simulink model "AdaptiveandRRTxBackstepping21a"  (R2022a)
settings: Solver=ode1  StartTime=0.0  StopTime=30  FixedStep=0.01  RelTol=1e-3  EnableMultiTasking=on
undefined symbols (not defined in the file): ux, uy
libraries: arduinolib x5, arduinosensorlib x1, mobileRoboticsLib x1
(part 1 of 2)
settings Model: NumberOfSteps=10  ExtModeTrigDuration=2  Creator=TR  LastModifiedBy=LabPC
settings DataIOCC: ReturnWorkspaceOutputs=off
settings OptimizationCC: EnhancedBackFolding=on  PassReuseOutputArgsAs=Individual arguments  ZeroExternalMemoryAtStartup=off  ZeroInternalMemoryAtStartup=off  MaxStackSize=64  OptimizeBlockOrder=speed  DifferentSizesBufferReuse=on  OptimizationCustomize=off  EfficientTunableParamExpr=on
settings DebuggingCC: ParameterTunabilityLossMsg=error  UnconnectedInputMsg=warning  UnconnectedOutputMsg=warning  UnconnectedLineMsg=warning
settings HardwareCC: ProdBitPerPointer=32  ProdBitPerSizeT=32  ProdBitPerPtrDiffT=32  ProdLargestAtomicInteger=Long  ProdLargestAtomicFloat=Double  ProdWordSize=32  ProdHWDeviceType=ARM Compatible->ARM Cortex
settings SFSimCC: MATLABDynamicMemAlloc=off
settings RTWCC: SystemTargetFile=ert.tlc  HardwareBoard=Arduino Due  TemplateMakefile=ert_default_tmf  Toolchain=Arduino ARM  BuildConfiguration=Faster Runs  DLArmComputeVersion=19.05
settings CodeAppCC: ForceParamTrailComments=on  IgnoreCustomStorageClasses=off  OperatorAnnotations=on  SimulinkDataObjDesc=on  SFDataObjDesc=on  InsertBlockDesc=on
settings ERTTargetCC: SupportContinuousTime=on  SupportVariableSizeSignals=on  ExtMode=on  ExtModeTransport=3  ExtModeStaticAlloc=on  ExtModeStaticAllocSize=24576  ExtModeMexFile=ext_xcp  ExtModeMexArgs=0 3 115200  ExtModeIntrfLevel=Level2 - Open

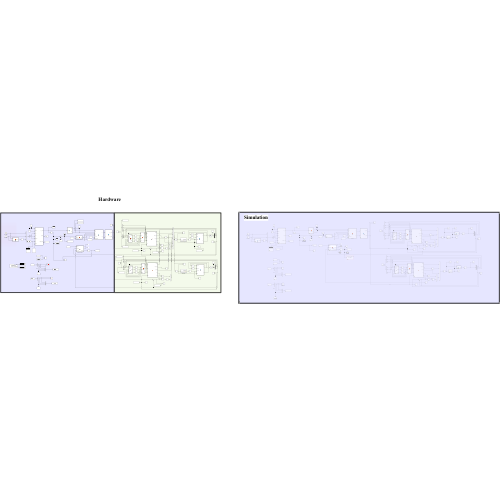
[thumbnail: Simulink's stored preview of the top-level diagram]
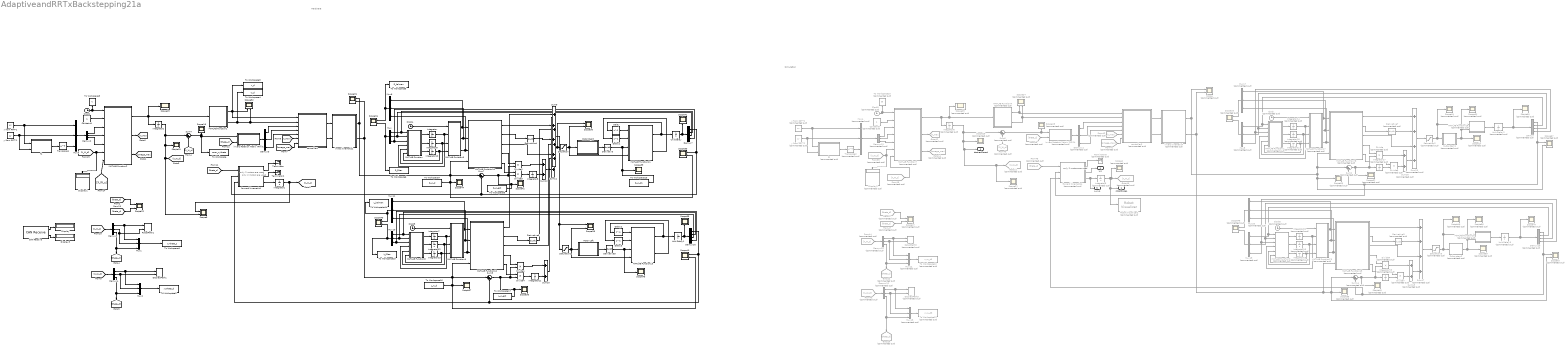
== system AdaptiveandRRTxBackstepping21a ==
  note: Hardware
  note: Simulation
  note: only 2 motors are used
  note: only 2 motors are used
  note: only 2 motors are used
  CAN Receive : arduinolib/CAN Receive  outputDataType=Raw data  identifierType=Standard (11-bit identifier)  messageId=100  msgLength=8  SampleTime=0.01  outputError=off  outputRemote=off
      settings: SourceProductBaseCode=ARDUINO
  Clock : Clock  Commented=on
  Clock1 : Clock
  Clock3 : Clock  Commented=on
  Clock4 : Clock
  Clock5 : Clock
  Clock6 : Clock  Commented=on
  Constant1 : Constant
  Constant2 : Constant  Commented=on
  Delay : Delay  DelayLength=1  InitialCondition=[0;0;0;0]
  Delay1 : Delay  DelayLength=1  InitialCondition=1e0*diag([10,1,30,10])
  Delay2 : Delay  DelayLength=1  InitialCondition=[0;0;0;0]
  Delay3 : Delay  DelayLength=1  InitialCondition=1e0*diag([10,1,30,10])
  Demux : Demux  Commented=on
  Demux{10..13} (4 alike) : Demux  Commented=on  Outputs=3
  Demux16 : Demux
  Demux{2..5} (4 alike) : Demux  Outputs=3
  Demux20 : Demux  Commented=on
  Demux7 : Demux
  Derivative{,4..6} (4 alike) : Derivative
  Derivative3 : Derivative  Commented=on
  Derivative7 : Derivative  Commented=on
  DesiredPath1 : Record  FileSettingsInternal="{\"entries\":[{\"content\":{\"excelSettings\":{\"content\":{},\"type\":\"Streamout.ExcelSettings\"}},\"type\":\"Streamout.FileSettingStorage\",\"uuid\":\"4478c04d-78d5-4c1c-a069-eeebce6a06e9\"}],\"packageUris\":[\"http://schema.mathworks.com/mf0/streamout_blocks/R2020a\"],\"version\":\"1.0\"}"  Layout=[1 1]  SignalsInternal="{\"entries\":[{\"content\":{\"signals\":[{\"content\":{\"blockPath\":[\"AdaptiveandRRTxBackstepping21a/DesiredPath1\"],\"channel\":[],\"dimensions\":[1],\"domain\":\"AdaptiveandRRTxBackstepping21a/DesiredPath1\",\"lineColor\":\"#a2142f\",\"plots\":[1],\"port\":1,\"sid\":[],\"signalID\":57046,\"signalName\":\"Demux4:1\"},\"type\":\"RecordBlkView.Signal\",\"uuid\":\"8b54ff27-c98d-4d9d-9907-af57662ca3f3\"},{\"content\":{\"blockPath\":[\"AdaptiveandRRTxBackstepping21a/DesiredPath1\"],\"channel\":[],\"dimensions\":[1],\"domain\":\"AdaptiveandRRTxBackstepping21a/DesiredPath1\",\"lineColor\":\"#139fff\",\"plots\":[1],\"port\":2,\"sid\":[],\"signalID\":57049,\"signalName\":\"Demux4:2\"},\"type\":\"RecordBlkView.Signal\",\"uuid\":\"d182928c-e909-4326-8931-a59e582ad6a8\"}]},\"type\":\"RecordBlkView.InputSignals\",\"uuid\":\"9f6ffbd3-a541-4e0a-a157-84b9438781ea\"}],\"packageUris\":[\"http://schema.mathworks.com/mf0/streamout_blocks/R2020a\"],\"version\":\"1.0\"}"  VisualizationBindings="{\"xyplotplugin\":{\"info\":[{\"series\":[{\"bindingParametersList\":[{\"parameter\":\"X-Axis\",\"signalID\":57046,\"signalName\":\"Demux4:1\"},{\"parameter\":\"Y-Axis\",\"signalID\":57049,\"signalName\":\"Demux4:2\"}],\"seriesID\":54754}],\"subplotID\":1}]}}"  CompatibilityTag=XY  st=-1
  DesiredPath3 : Record  Commented=on  FileSettingsInternal="{\"entries\":[{\"content\":{\"excelSettings\":{\"content\":{},\"type\":\"Streamout.ExcelSettings\"}},\"type\":\"Streamout.FileSettingStorage\",\"uuid\":\"5e9f582f-be01-4ee5-aef2-fee70209bf0f\"}],\"packageUris\":[\"http://schema.mathworks.com/mf0/streamout_blocks/R2020a\"],\"version\":\"1.0\"}"  Layout=[1 1]  SignalsInternal="{\"entries\":[{\"content\":{\"signals\":[{\"content\":{\"blockPath\":[\"AdaptiveandRRTxBackstepping21a/DesiredPath3\"],\"channel\":[],\"dimensions\":[1],\"domain\":\"AdaptiveandRRTxBackstepping21a/DesiredPath3\",\"lineColor\":\"#a2142f\",\"plots\":[1],\"port\":1,\"sid\":[],\"signalID\":57038,\"signalName\":\"XY Graph:1\"},\"type\":\"RecordBlkView.Signal\",\"uuid\":\"5ec44264-e469-460e-9c8e-a5441ec41171\"},{\"content\":{\"blockPath\":[\"AdaptiveandRRTxBackstepping21a/DesiredPath3\"],\"channel\":[],\"dimensions\":[1],\"domain\":\"AdaptiveandRRTxBackstepping21a/DesiredPath3\",\"lineColor\":\"#139fff\",\"plots\":[1],\"port\":2,\"sid\":[],\"signalID\":57041,\"signalName\":\"XY Graph:2\"},\"type\":\"RecordBlkView.Signal\",\"uuid\":\"ca682f9e-4f20-4675-ba71-c6bfc3bf3438\"}]},\"type\":\"RecordBlkView.InputSignals\",\"uuid\":\"5794ffc7-f7ba-41dc-b1e7-413d37048635\"}],\"packageUris\":[\"http://schema.mathworks.com/mf0/streamout_blocks/R2020a\"],\"version\":\"1.0\"}"  VisualizationBindings="{\"xyplotplugin\":{\"info\":[{\"series\":[{\"bindingParametersList\":[{\"parameter\":\"X-Axis\",\"signalID\":57038,\"signalName\":\"XY Graph:1\"},{\"parameter\":\"Y-Axis\",\"signalID\":57041,\"signalName\":\"XY Graph:2\"}],\"seriesID\":2614}],\"subplotID\":1}]}}"  CompatibilityTag=XY  st=-1
  Display : Display
  Display1 : Display
  Display2 : Display  Commented=on
  Display3 : Display
  Divide{,5..7} (4 alike) : Product  Commented=on  Inputs=**
  Divide{1..4} (4 alike) : Product  Inputs=**
  From15 : From  Commented=on  GotoTag=X_W_c
  From35 : From  Commented=on  GotoTag=X_W_d
  From37 : From  Commented=on  GotoTag=theta_d
  From40 : From  Commented=on  GotoTag=X_W_c
  From41 : From  Commented=on  GotoTag=omega_max
  From42 : From  Commented=on  GotoTag=V_max
  From43 : From  Commented=on  GotoTag=X_W_d
  From44 : From  Commented=on  GotoTag=X_W_c
  From45 : From  Commented=on  GotoTag=theta_c
  From46 : From  Commented=on  GotoTag=theta_c
  From47 : From  Commented=on  GotoTag=theta_c
  Goto12 : Goto  Commented=on  GotoTag=V_max
  Goto14 : Goto  Commented=on  GotoTag=omega_max
  Goto16 : Goto  Commented=on  GotoTag=X_W_c
  Goto21 : Goto  Commented=on  GotoTag=X_W_d
  Goto22 : Goto  Commented=on  GotoTag=theta_c
  Goto23 : Goto  Commented=on  GotoTag=theta_d
  Integrator : Integrator  InitialCondition=28.37
  Integrator1 : Integrator  InitialCondition=[0;0;0]
  Integrator10 : Integrator  InitialCondition=5.750
  Integrator11 : Integrator
  Integrator12 : Integrator  InitialCondition=17.26
  Integrator13 : Integrator  InitialCondition=6.776
  Integrator14 : Integrator  Commented=on  InitialCondition=28.37
  Integrator15 : Integrator  Commented=on  InitialCondition=17.26
  Integrator16 : Integrator  Commented=on  InitialCondition=6.776
  Integrator17 : Integrator  Commented=on
  Integrator18 : Integrator  Commented=on  InitialCondition=19.15
  Integrator2 : Integrator
  Integrator21 : Integrator  Commented=on  InitialCondition=5.75
  Integrator22 : Integrator  Commented=on  InitialCondition=26.63
  Integrator23 : Integrator  Commented=on
  Integrator5 : Integrator  Commented=on  InitialCondition=[0;0;0]
  Integrator6 : Integrator  Commented=on
  Integrator7 : Integrator  InitialCondition=26.63
  Integrator8 : Integrator
  Integrator9 : Integrator  InitialCondition=19.15
  MATLAB Function : MATLAB Function  TreatAsAtomicUnit=on
  MATLAB Function1 : MATLAB Function  TreatAsAtomicUnit=on
  MATLAB Function10 : MATLAB Function  TreatAsAtomicUnit=on
  MATLAB Function11 : MATLAB Function  TreatAsAtomicUnit=on
  MATLAB Function12 : MATLAB Function  TreatAsAtomicUnit=on
  MATLAB Function13 : MATLAB Function  TreatAsAtomicUnit=on
  MATLAB Function14 : MATLAB Function  Commented=on  TreatAsAtomicUnit=on
  MATLAB Function15 : MATLAB Function  Commented=on  TreatAsAtomicUnit=on
  MATLAB Function16 : MATLAB Function  Commented=on  TreatAsAtomicUnit=on
  MATLAB Function17 : MATLAB Function  Commented=on  TreatAsAtomicUnit=on
  MATLAB Function18 : MATLAB Function  Commented=on  TreatAsAtomicUnit=on
  MATLAB Function19 : MATLAB Function  Commented=on  TreatAsAtomicUnit=on
  MATLAB Function2 : MATLAB Function  TreatAsAtomicUnit=on
  MATLAB Function22 : MATLAB Function  Commented=on  TreatAsAtomicUnit=on
  MATLAB Function23 : MATLAB Function  Commented=on  TreatAsAtomicUnit=on
  MATLAB Function5 : MATLAB Function  TreatAsAtomicUnit=on
  MATLAB Function6 : MATLAB Function  Commented=on  TreatAsAtomicUnit=on
  MATLAB Function7 : MATLAB Function  Commented=on  TreatAsAtomicUnit=on
  MATLAB Function8 : MATLAB Function  TreatAsAtomicUnit=on
  MATLAB Function9 : MATLAB Function  TreatAsAtomicUnit=on
  Motor Left : Subsystem
  Motor Right : Subsystem
  Mux{,1..2,8..11} (7 alike) : Mux  Inputs=3
  Mux{4..5,12..13,17,19..20} (7 alike) : Mux  Commented=on  Inputs=3
  Robot Visualizer1 : mobileRoboticsLib/Environments/Robot Visualizer  Priority=99  Commented=on  robotRadius=0.22  showTrajectory=on  hasWaypoints=off  hasLidar=off  sensorOffset=scanSensorOffset  scanAngles=scanAngles  hasObjDetector=off  objDetectorOffset=[ 0, 0 ]  objDetectorAngle=0  objDetectorFOV=0  objDetectorMaxRange=0  objectColors=0  objectMarkers='s'
  RobotPath1 : Record  FileSettingsInternal="{\"entries\":[{\"content\":{\"excelSettings\":{\"content\":{},\"type\":\"Streamout.ExcelSettings\"}},\"type\":\"Streamout.FileSettingStorage\",\"uuid\":\"0ff43101-e007-4439-8427-ec14aa2ad80f\"}],\"packageUris\":[\"http://schema.mathworks.com/mf0/streamout_blocks/R2020a\"],\"version\":\"1.0\"}"  Layout=[1 1]  SignalsInternal="{\"entries\":[{\"content\":{\"signals\":[{\"content\":{\"blockPath\":[\"AdaptiveandRRTxBackstepping21a/RobotPath1\"],\"channel\":[],\"dimensions\":[1],\"domain\":\"AdaptiveandRRTxBackstepping21a/RobotPath1\",\"lineColor\":\"#a2142f\",\"plots\":[1],\"port\":1,\"sid\":[],\"signalID\":57030,\"signalName\":\"x_c\"},\"type\":\"RecordBlkView.Signal\",\"uuid\":\"07d52e62-8ab4-4c53-9fa3-f17bd603cef6\"},{\"content\":{\"blockPath\":[\"AdaptiveandRRTxBackstepping21a/RobotPath1\"],\"channel\":[],\"dimensions\":[1],\"domain\":\"AdaptiveandRRTxBackstepping21a/RobotPath1\",\"lineColor\":\"#139fff\",\"plots\":[1],\"port\":2,\"sid\":[],\"signalID\":57033,\"signalName\":\"y_c\"},\"type\":\"RecordBlkView.Signal\",\"uuid\":\"97726e5f-6405-4899-84cb-06a72cfc2d61\"}]},\"type\":\"RecordBlkView.InputSignals\",\"uuid\":\"38ea1586-2402-407b-8988-e549c318f5ad\"}],\"packageUris\":[\"http://schema.mathworks.com/mf0/streamout_blocks/R2020a\"],\"version\":\"1.0\"}"  VisualizationBindings="{\"xyplotplugin\":{\"info\":[{\"series\":[{\"bindingParametersList\":[{\"parameter\":\"X-Axis\",\"signalID\":57030,\"signalName\":\"x_c\"},{\"parameter\":\"Y-Axis\",\"signalID\":57033,\"signalName\":\"y_c\"}],\"seriesID\":57420}],\"subplotID\":1}]}}"  CompatibilityTag=XY  st=-1
  RobotPath3 : Record  Commented=on  FileSettingsInternal="{\"entries\":[{\"content\":{\"excelSettings\":{\"content\":{},\"type\":\"Streamout.ExcelSettings\"}},\"type\":\"Streamout.FileSettingStorage\",\"uuid\":\"6211d518-7cd9-4385-8e1e-1901f1a620c4\"}],\"packageUris\":[\"http://schema.mathworks.com/mf0/streamout_blocks/R2020a\"],\"version\":\"1.0\"}"  Layout=[1 1]  SignalsInternal="{\"entries\":[{\"content\":{\"signals\":[{\"content\":{\"blockPath\":[\"AdaptiveandRRTxBackstepping21a/RobotPath3\"],\"channel\":[],\"dimensions\":[1],\"domain\":\"AdaptiveandRRTxBackstepping21a/RobotPath3\",\"lineColor\":\"#a2142f\",\"plots\":[1],\"port\":1,\"sid\":[],\"signalID\":57022,\"signalName\":\"XY Graph:1\"},\"type\":\"RecordBlkView.Signal\",\"uuid\":\"6d308a3b-99d3-4536-8b9f-580f0f8d7449\"},{\"content\":{\"blockPath\":[\"AdaptiveandRRTxBackstepping21a/RobotPath3\"],\"channel\":[],\"dimensions\":[1],\"domain\":\"AdaptiveandRRTxBackstepping21a/RobotPath3\",\"lineColor\":\"#139fff\",\"plots\":[1],\"port\":2,\"sid\":[],\"signalID\":57025,\"signalName\":\"XY Graph:2\"},\"type\":\"RecordBlkView.Signal\",\"uuid\":\"215d46f4-e3f5-46fc-8db7-d861b213b18e\"}]},\"type\":\"RecordBlkView.InputSignals\",\"uuid\":\"501962c1-ec9d-432a-b496-bf00d34232ec\"}],\"packageUris\":[\"http://schema.mathworks.com/mf0/streamout_blocks/R2020a\"],\"version\":\"1.0\"}"  VisualizationBindings="{\"xyplotplugin\":{\"info\":[{\"series\":[{\"bindingParametersList\":[{\"parameter\":\"X-Axis\",\"signalID\":57022,\"signalName\":\"XY Graph:1\"},{\"parameter\":\"Y-Axis\",\"signalID\":57025,\"signalName\":\"XY Graph:2\"}],\"seriesID\":23653}],\"subplotID\":1}]}}"  CompatibilityTag=XY  st=-1
  Saturation : Saturate  UpperLimit=23  LowerLimit=-23
  Saturation1 : Saturate  UpperLimit=23  LowerLimit=-23
  Saturation2 : Saturate  Commented=on  UpperLimit=23  LowerLimit=-23
  Saturation3 : Saturate  Commented=on  UpperLimit=23  LowerLimit=-23
  Scope{,20..21,24,46,61..62} (7 alike) : Scope  Commented=on  NumInputPorts=2
  Scope{15,18..19,35..37,39,41..42,44..45} (11 alike) : Scope
  Scope{2,17,23,25,28..29,47..49,55..56,59..60,63..66} (17 alike) : Scope  Commented=on
  Scope{8,22,30..34,38,40,43} (10 alike) : Scope  NumInputPorts=2
  Subsystem1 : Subsystem  Commented=on
  Subsystem2 : Subsystem  Commented=on
  Sum10 : Sum
  Sum11 : Sum  Inputs=++++
  Sum12 : Sum
  Sum13 : Sum  Commented=on  Inputs=++++
  Sum14 : Sum  Commented=on  Inputs=|+-
  Sum16 : Sum  Commented=on
  Sum17 : Sum  Commented=on  Inputs=++++
  Sum18 : Sum  Commented=on
  Sum2 : Sum  Commented=on  Inputs=|+-
  Sum4 : Sum  Inputs=|+-
  Sum6 : Sum  Commented=on  Inputs=|+-
  Sum7 : Sum  Inputs=|+-
  Sum8 : Sum  Inputs=|+-
  Sum9 : Sum  Inputs=++++
  Terminator : Terminator
  Terminator1 : Terminator
  Terminator3 : Terminator  Commented=on
  To Workspace : ToWorkspace  VariableName=error_xytheta  SaveFormat=Structure With Time  SampleTime=-1
  To Workspace1 : ToWorkspace  VariableName=xytheta_c  SaveFormat=Structure With Time  SampleTime=-1
  To Workspace10 : ToWorkspace  Commented=on  VariableName=t3  SampleTime=-1
  To Workspace11 : ToWorkspace  Commented=on  VariableName=xyw_d3  SaveFormat=Timeseries  SampleTime=-1
  To Workspace12 : ToWorkspace  Commented=on  VariableName=xyw_c3  SaveFormat=Timeseries  SampleTime=-1
  To Workspace13 : ToWorkspace  VariableName=R_w_d1  SaveFormat=Structure With Time  SampleTime=-1
  To Workspace14 : ToWorkspace  VariableName=L_kalman  SaveFormat=Structure With Time  SampleTime=-1
  To Workspace15 : ToWorkspace  VariableName=L_filter  SaveFormat=Structure With Time  SampleTime=-1
  To Workspace16 : ToWorkspace  VariableName=L_w_d  SaveFormat=Structure With Time  SampleTime=-1
  To Workspace17 : ToWorkspace  VariableName=L_w_est  SaveFormat=Structure With Time  SampleTime=-1
  To Workspace2 : ToWorkspace  VariableName=xytheta_d  SaveFormat=Structure With Time  SampleTime=-1
  To Workspace3 : ToWorkspace  VariableName=v_d  SaveFormat=Structure With Time  SampleTime=-1
  To Workspace4 : ToWorkspace  VariableName=w_d  SaveFormat=Structure With Time  SampleTime=-1
  To Workspace5 : ToWorkspace  VariableName=R_kalman  SaveFormat=Structure With Time  SampleTime=-1
  To Workspace6 : ToWorkspace  VariableName=R_filter  SaveFormat=Structure With Time  SampleTime=-1
  To Workspace7 : ToWorkspace  VariableName=R_w_d  SaveFormat=Structure With Time  SampleTime=-1
  To Workspace8 : ToWorkspace  VariableName=R_w_est  SaveFormat=Structure With Time  SampleTime=-1
  To Workspace9 : ToWorkspace  VariableName=t  SampleTime=-1
  Transpose1 : Math  Operator=transpose
  Transpose2 : Math  Commented=on  Operator=transpose
  Unit Delay : UnitDelay  SampleTime=-1  HasFrameUpgradeWarning=on
  Unit Delay1 : UnitDelay  SampleTime=-1  HasFrameUpgradeWarning=on
  Unit Delay2 : UnitDelay  Commented=on  SampleTime=-1  HasFrameUpgradeWarning=on
  Unit Delay3 : UnitDelay  Commented=on  SampleTime=-1  HasFrameUpgradeWarning=on
  controller1 : MATLAB Function  TreatAsAtomicUnit=on
  controller3 : MATLAB Function  Commented=on  TreatAsAtomicUnit=on
  f1 : MATLAB Function  TreatAsAtomicUnit=on
  f2 : MATLAB Function  Commented=on  TreatAsAtomicUnit=on
  forward kinematic1 : MATLAB Function  TreatAsAtomicUnit=on
  forward kinematic4 : MATLAB Function  Commented=on  TreatAsAtomicUnit=on
  invers Rotation Matrix (R(fi))1 : MATLAB Function  TreatAsAtomicUnit=on
  invers Rotation Matrix (R(fi))4 : MATLAB Function  Commented=on  TreatAsAtomicUnit=on
  invers kinematic1 : MATLAB Function  TreatAsAtomicUnit=on
  invers kinematic4 : MATLAB Function  Commented=on  TreatAsAtomicUnit=on
  x from RRT*1 : Constant  Value=ux
  x from RRT*2 : Constant  Commented=on  Value=ux
  y from RRT*1 : Constant  Value=uy
  y from RRT*2 : Constant  Commented=on  Value=uy
  robotPose4 : Outport
  desiredPose4 : Outport  Port=2
  v_xy4 : Outport  Port=3
  w4 : Outport  Port=4
  wires:
  Demux11/1 -> controller3/3(e1)
  invers Rotation Matrix (R(fi))4/1(e_R) -> Demux11/1
  From41/1 -> controller3/7(omega_max)
  Mux4/1 -> Demux10/1
  Demux10/1 -> MATLAB Function7/3(x_d)
  MATLAB Function7/3(omega_max) -> Goto14/1
  From42/1 -> controller3/6(V_max)
  Demux10/3 -> MATLAB Function7/5(theta_d)
  MATLAB Function7/2(V_max) -> Goto12/1
  From40/1 -> Sum6/2  "xyd_c"
  Demux13/3 -> Mux12/3, Goto22/1  "theta_c"
  From37/1 -> Scope21/1
  controller3/2(w_c) -> invers kinematic4/2(w)
  MATLAB Function6/1(v_d) -> Scope24/1, controller3/1(v_d)
  Demux12/2 -> Mux13/2, DesiredPath3/2
  Demux10/2 -> MATLAB Function7/4(y_d)
  Integrator5/1 -> Scope2/1, Goto16/1, Robot Visualizer1/1, robotPose4/1
  Sum6/1 -> invers Rotation Matrix (R(fi))4/1(e_w), Scope28/1
  Demux12/1 -> Mux13/1, DesiredPath3/1
  y from RRT*2/1 -> Mux4/2, f2/2(y_d)
  Transpose2/1 -> Mux4/3
  Demux11/3 -> controller3/5(e3)
  Clock3/1 -> MATLAB Function7/1(t), To Workspace10/1
  Demux11/2 -> controller3/4(e2)
  From44/1 -> Demux13/1
  Mux13/1 -> To Workspace11/1
  Integrator6/1 -> Goto21/1, Scope23/1, desiredPose4/1, Scope29/1, Sum6/1  "xyw_d"
  Constant2/1 -> MATLAB Function7/2(route)
  forward kinematic4/2(w) -> w4/1
  From45/1 -> forward kinematic4/1(theta_c)
  x from RRT*2/1 -> f2/1(x_d), Mux4/1
  MATLAB Function7/1(X_r_dot) -> Scope25/1, MATLAB Function6/1(Xd_dot), Integrator6/1
  From35/1 -> Display2/1, MATLAB Function7/6(X)
  forward kinematic4/3(X_W_dot) -> Integrator5/1, v_xy4/1
  forward kinematic4/1(v) -> Terminator3/1
  From47/1 -> Scope21/2
  Demux13/2 -> Mux12/2, RobotPath3/2  "y_c"
  Demux13/1 -> Mux12/1, RobotPath3/1  "x_c"
  From46/1 -> invers Rotation Matrix (R(fi))4/2(theta_c)
  From43/1 -> Demux12/1
  Demux12/3 -> Goto23/1, Mux13/3  "theta_d"
  controller3/1(v_c) -> invers kinematic4/1(v)
  MATLAB Function6/2(w_d) -> controller3/2(w_d), Scope24/2
  f2/1(theta_d) -> Transpose2/1
  Mux12/1 -> To Workspace12/1
  From15/1 -> MATLAB Function7/7(X_W_c)
  Sum4/1 -> To Workspace/1, invers Rotation Matrix (R(fi))1/1(e_w), Scope18/1
  Demux2/1 -> MATLAB Function2/3(x_d)
  invers Rotation Matrix (R(fi))1/1(e_R) -> Demux3/1
  Demux5/1 -> Mux1/1, RobotPath1/1  "x_c"
  Demux4/2 -> DesiredPath1/2, Mux2/2
  [omega_max] -> controller1/7(omega_max)
  MATLAB Function2/3(omega_max) -> [omega_max]
  [theta_c] -> forward kinematic1/1(theta_c)
  [theta_d] -> Scope22/1
  Demux5/3 -> [theta_c], Mux1/3  "theta_c"
  controller1/2(w_c) -> invers kinematic1/2(w)
  Demux7/1 -> Sum7/2, forward kinematic1/2(fi_R_dot), Scope33/1
  Demux2/3 -> MATLAB Function2/5(theta_d)
  Integrator1/1 -> Scope8/1, [X_W_c]
  Demux4/1 -> DesiredPath1/1, Mux2/1
  MATLAB Function2/2(V_max) -> [V_max]
  Demux3/3 -> controller1/5(e3)
  [X_W_c] -> Sum4/2  "xyd_c"
  Mux9/1 -> Demux2/1
  Demux3/1 -> controller1/3(e1)
  Constant1/1 -> MATLAB Function2/2(route)
  forward kinematic1/1(v) -> Terminator/1
  forward kinematic1/3(X_W_dot) -> Integrator1/1
  MATLAB Function1/2(w_d) -> controller1/2(w_d), Scope32/2, To Workspace4/1
  x from RRT*1/1 -> Mux9/1, f1/1(x_d)
  MATLAB Function1/1(v_d) -> Scope32/1, To Workspace3/1, controller1/1(v_d)
  f1/1(theta_d) -> Transpose1/1
  Mux2/1 -> To Workspace2/1
  MATLAB Function2/1(X_r_dot) -> Scope15/1, Integrator2/1, MATLAB Function1/1(Xd_dot)
  Clock1/1 -> To Workspace9/1, MATLAB Function2/1(t)
  Demux3/2 -> controller1/4(e2)
  [V_max] -> controller1/6(V_max)
  Demux2/2 -> MATLAB Function2/4(y_d)
  forward kinematic1/2(w) -> Terminator1/1
  Mux1/1 -> To Workspace1/1
  [theta_c] -> Scope22/2
  Integrator2/1 -> Scope8/2, [X_W_d], Scope19/1, Sum4/1  "xyw_d"
  [X_W_c] -> MATLAB Function2/7(X_W_c)
  [X_W_d] -> Display1/1, MATLAB Function2/6(X)
  [theta_c] -> invers Rotation Matrix (R(fi))1/2(theta_c)
  y from RRT*1/1 -> f1/2(y_d), Mux9/2
  Demux4/3 -> Mux2/3, [theta_d]  "theta_d"
  controller1/1(v_c) -> invers kinematic1/1(v)
  Demux5/2 -> RobotPath1/2, Mux1/2  "y_c"
  [X_W_d] -> Demux4/1
  Transpose1/1 -> Mux9/3
  [X_W_c] -> Demux5/1
  MATLAB Function10/3(a_on_b) -> Sum11/3
  Derivative5/1 -> Scope45/1, MATLAB Function13/3(y_true)
  MATLAB Function9/1(a) -> Mux11/1, MATLAB Function12/1(a)
  Integrator7/1 -> MATLAB Function9/2(a_nw), MATLAB Function8/4(a)
  Derivative/1 -> To Workspace13/1, Scope39/1, MATLAB Function11/3(y_true)
  MATLAB Function5/1(a) -> Mux8/1, MATLAB Function10/1(a)
  Clock5/1 -> MATLAB Function9/1(t)
  Integrator12/1 -> MATLAB Function8/5(b), MATLAB Function9/3(b_nw)
  Divide1/1 -> Sum10/1
  Sum10/1 -> Sum9/4
  MATLAB Function12/5(ki) -> Divide4/1
  Saturation/1 -> MATLAB Function11/4(uk), Motor Right/1(u), Scope30/2
  invers kinematic1/1(fi_R_dot) -> MATLAB Function10/4(w), Scope44/1, To Workspace7/1, Scope33/2, Sum7/1, Scope31/1
  Sum9/1 -> Saturation1/1, Scope38/1
  Unit Delay1/1 -> Demux16/1, Scope35/1
  Demux7/3 -> MATLAB Function/2(b_hat), Mux/2
  MATLAB Function12/1(comp) -> Sum9/1
  MATLAB Function13/1(x) -> Delay2/1, Unit Delay1/1
  Demux16/3 -> MATLAB Function8/2(b_hat), Mux10/2
  invers kinematic1/2(fi_L_dot) -> Scope31/2, Scope40/2, To Workspace16/1, Scope37/1, MATLAB Function12/4(w), Sum8/1
  Motor Right/1(outGearBox) -> Derivative/1
  Demux16/2 -> MATLAB Function8/1(a_hat), Mux10/1
  MATLAB Function8/2(b_dot) -> Integrator12/1
  Delay2/1 -> MATLAB Function13/1(x_pre)
  Sum8/1 -> To Workspace17/1, Scope36/1, Divide1/2, Divide4/2
  Derivative6/1 -> Sum9/2  "wd_dot"
  Mux11/1 -> Scope43/1, To Workspace14/1
  MATLAB Function10/2(one_on_b) -> Derivative4/1
  Divide4/1 -> Integrator11/1
  Saturation1/1 -> Motor Left/1(u), MATLAB Function13/4(uk), Scope38/2
  Integrator11/1 -> Sum10/2
  Integrator13/1 -> MATLAB Function9/4(c_nw), MATLAB Function8/6(c)
  MATLAB Function12/2(one_on_b) -> Derivative6/1
  MATLAB Function13/2(P) -> Delay3/1
  Mux10/1 -> Scope43/2, To Workspace15/1
  MATLAB Function12/3(a_on_b) -> Sum9/3
  Divide2/1 -> Sum12/1
  Demux16/4 -> MATLAB Function8/3(c_hat), Mux10/3
  MATLAB Function9/3(c) -> Mux11/3, MATLAB Function12/3(c)
  Derivative4/1 -> Sum11/2  "wd_dot"
  MATLAB Function11/1(x) -> Delay/1, Unit Delay/1
  MATLAB Function5/2(b) -> Mux8/2, MATLAB Function10/2(b)
  MATLAB Function5/3(c) -> Mux8/3, MATLAB Function10/3(c)
  Demux7/4 -> MATLAB Function/3(c_hat), Mux/3
  MATLAB Function10/4(kp) -> Divide2/1
  Integrator8/1 -> Sum12/2
  Sum11/1 -> Scope30/1, Saturation/1
  Delay3/1 -> MATLAB Function13/2(P_pre)
  Unit Delay/1 -> Demux7/1, Scope41/1
  MATLAB Function10/1(comp) -> Sum11/1
  Mux8/1 -> Scope34/1, To Workspace5/1
  Divide3/1 -> Integrator8/1
  Demux7/2 -> MATLAB Function/1(a_hat), Mux/1
  Integrator9/1 -> MATLAB Function/5(b), MATLAB Function5/3(b_nw)
  MATLAB Function9/2(b) -> Mux11/2, MATLAB Function12/2(b)
  MATLAB Function12/4(kp) -> Divide1/1
  Mux/1 -> To Workspace6/1, Scope34/2
  MATLAB Function10/5(ki) -> Divide3/1
  Clock4/1 -> MATLAB Function5/1(t)
  Delay1/1 -> MATLAB Function11/2(P_pre)
  MATLAB Function/2(b_dot) -> Integrator9/1
  MATLAB Function/3(c_dot) -> Integrator10/1
  MATLAB Function8/3(c_dot) -> Integrator13/1
  MATLAB Function8/1(a_dot) -> Integrator7/1
  Integrator/1 -> MATLAB Function5/2(a_nw), MATLAB Function/4(a)
  Sum7/1 -> To Workspace8/1, Scope42/1, Divide2/2, Divide3/2
  Delay/1 -> MATLAB Function11/1(x_pre)
  Sum12/1 -> Sum11/4
  MATLAB Function/1(a_dot) -> Integrator/1
  Motor Left/1(outGearBox) -> Derivative5/1
  Integrator10/1 -> MATLAB Function5/4(c_nw), MATLAB Function/6(c)
  MATLAB Function11/2(P) -> Delay1/1
  Demux16/1 -> Sum8/2, forward kinematic1/3(fi_L_dot), Scope40/1
  Integrator15/1 -> MATLAB Function22/5(b), MATLAB Function23/3(b_nw)
  MATLAB Function15/2(one_on_b) -> Derivative3/1
  Demux20/2 -> Mux19/1, MATLAB Function22/1(a_hat)
  Integrator22/1 -> MATLAB Function23/2(a_nw), MATLAB Function22/4(a)
  MATLAB Function22/3(c_dot) -> Integrator16/1
  Mux19/1 -> Scope46/2
  Sum14/1 -> Scope48/1, Integrator23/1, Divide6/2
  MATLAB Function22/1(a_dot) -> Integrator22/1
  MATLAB Function16/1(x_est) -> Unit Delay3/1
  MATLAB Function15/4(kp) -> Divide6/1
  MATLAB Function23/2(b) -> Mux20/2, MATLAB Function15/2(b)
  Sum17/1 -> Saturation3/1
  Integrator16/1 -> MATLAB Function23/4(c_nw), MATLAB Function22/6(c)
  MATLAB Function22/2(b_dot) -> Integrator15/1
  Integrator23/1 -> Divide7/2
  Sum18/1 -> Sum17/4
  MATLAB Function15/1(comp) -> Sum17/1
  Clock6/1 -> MATLAB Function23/1(t)
  Subsystem2/1(Output) -> Scope59/1, Scope56/1, MATLAB Function16/2(y_true)
  MATLAB Function15/3(a_on_b) -> Sum17/3
  Derivative3/1 -> Sum17/2  "wd_dot"
  Unit Delay3/1 -> Scope47/1, Demux20/1
  MATLAB Function23/3(c) -> Mux20/3, MATLAB Function15/3(c)
  Divide6/1 -> Sum18/1
  MATLAB Function23/1(a) -> Mux20/1, MATLAB Function15/1(a)
  Demux20/3 -> Mux19/2, MATLAB Function22/2(b_hat)
  Divide7/1 -> Sum18/2
  MATLAB Function15/5(ki) -> Divide7/1
  Demux20/1 -> forward kinematic4/3(fi_L_dot), Sum14/2, Scope61/1
  invers kinematic4/2(fi_L_dot) -> Scope/2, MATLAB Function15/4(w), Scope61/2, Sum14/1, Scope55/1  "wd_L"
  Saturation3/1 -> Subsystem2/1(va), Scope49/1, MATLAB Function16/1(uk)
  Mux20/1 -> Scope46/1
  Demux20/4 -> Mux19/3, MATLAB Function22/3(c_hat)
  MATLAB Function18/1(comp) -> Sum13/1
  Mux5/1 -> Scope20/2
  Saturation2/1 -> Subsystem1/1(va), Scope64/1, MATLAB Function19/1(uk)
  Demux/1 -> Scope62/1, forward kinematic4/2(fi_R_dot), Sum2/2
  Mux17/1 -> Scope20/1
  MATLAB Function19/1(x_est) -> Unit Delay2/1
  MATLAB Function17/3(c) -> Mux17/3, MATLAB Function18/3(c)
  Demux/2 -> Mux5/1, MATLAB Function14/1(a_hat)
  Sum2/1 -> Scope63/1, Integrator17/1, Divide/2
  MATLAB Function18/3(a_on_b) -> Sum13/3
  MATLAB Function18/5(ki) -> Divide5/1
  MATLAB Function18/2(one_on_b) -> Derivative7/1
  MATLAB Function17/2(b) -> Mux17/2, MATLAB Function18/2(b)
  Integrator17/1 -> Divide5/2
  Sum13/1 -> Saturation2/1
  Sum16/1 -> Sum13/4
  Integrator21/1 -> MATLAB Function17/4(c_nw), MATLAB Function14/6(c)
  Demux/3 -> Mux5/2, MATLAB Function14/2(b_hat)
  Integrator18/1 -> MATLAB Function14/5(b), MATLAB Function17/3(b_nw)
  invers kinematic4/1(fi_R_dot) -> Sum2/1, MATLAB Function18/4(w), Scope62/2, Scope65/1, Scope/1  "wd_R"
  MATLAB Function14/1(a_dot) -> Integrator14/1
  MATLAB Function14/2(b_dot) -> Integrator18/1
  Subsystem1/1(Output) -> Scope17/1, Scope66/1, MATLAB Function19/2(y_true)
  MATLAB Function18/4(kp) -> Divide/1
  Demux/4 -> Mux5/3, MATLAB Function14/3(c_hat)
  Clock/1 -> MATLAB Function17/1(t)
  MATLAB Function14/3(c_dot) -> Integrator21/1
  Divide/1 -> Sum16/1
  Unit Delay2/1 -> Scope60/1, Demux/1
  Derivative7/1 -> Sum13/2  "wd_dot"
  Integrator14/1 -> MATLAB Function17/2(a_nw), MATLAB Function14/4(a)
  MATLAB Function17/1(a) -> Mux17/1, MATLAB Function18/1(a)
  Divide5/1 -> Sum16/2
  CAN Receive/1 -> Display/1
  CAN Receive/2 -> Display3/1

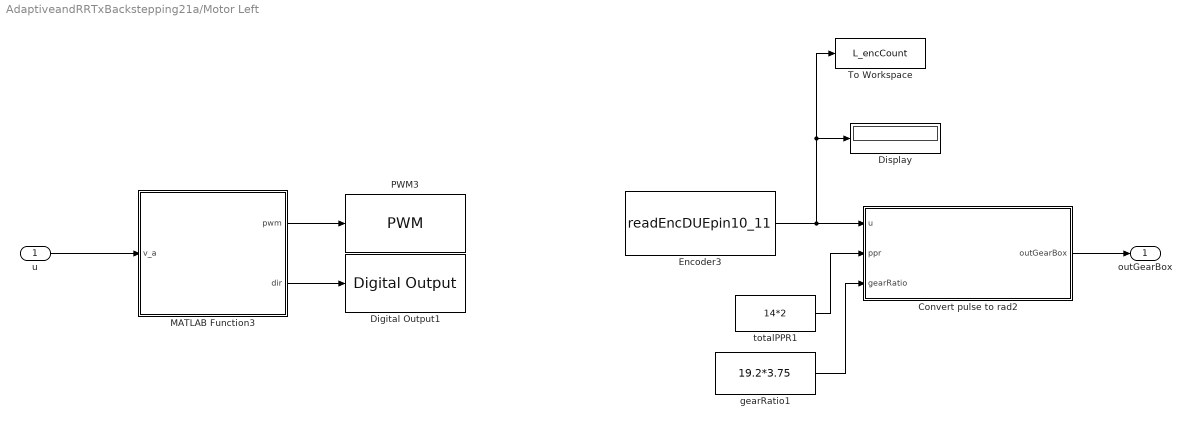
== system AdaptiveandRRTxBackstepping21a/Motor Left ==
  u : Inport
  Convert pulse to rad2 : MATLAB Function  TreatAsAtomicUnit=on
  Digital Output1 : arduinolib/Digital Output  pinNumber=4  Direction=output  blockPlatform=arduino
  Display : Display
  Encoder3 : S-Function  InitFcn=try, set_param(gcb,'FunctionName','readEncDUEpin10_11'), end  FunctionName=readEncDUEpin10_11  SFunctionModules=readEncDUEpin10_11_wrapper  SFunctionDeploymentMode=off  EnableBusSupport=off  mask(S-Function Builder){}
      mask help: Simulink:masks:SFunctionBuilder_MD
      mask init:
      | val = [[.9  0.75 0.75 1 1 .9 .9 1]',[1 1 0.75 0.75 .9 .9 1 .9]'];try , sys = get_param(gcb,'SfunBuilderFcnName');if isempty(sys), sys = get_param(gcb,'FunctionName'); end,catch, sys = get_param(gcb,'FunctionName'); end
      settings: CopyFcn=set_param(gcbh,'LinkStatus','none')  PreSaveFcn=try, set_param(gcb,'FunctionName','readEncDUEpin10_11'), end  OpenFcn=sfunctionwizard(gcbh)
      mask Display:
      | plot(val(:,1),val(:,2))
      | disp(sys)
      | port_label('output',1,'countt')
  MATLAB Function3 : MATLAB Function  TreatAsAtomicUnit=on
  PWM3 : arduinolib/PWM  pinNumber=5  frequencyType=Default  desiredFrequency=490.2  achievableFrequency=490.2
  To Workspace : ToWorkspace  VariableName=L_encCount  SaveFormat=Timeseries  SampleTime=-1
  gearRatio1 : Constant  Value=19.2*3.75
  totalPPR1 : Constant  Value=14*2
  outGearBox : Outport
  wires:
  Encoder3/1 -> Convert pulse to rad2/1(u), Display/1, To Workspace/1
  MATLAB Function3/2(dir) -> Digital Output1/1
  MATLAB Function3/1(pwm) -> PWM3/1
  u/1 -> MATLAB Function3/1(v_a)
  gearRatio1/1 -> Convert pulse to rad2/3(gearRatio)
  totalPPR1/1 -> Convert pulse to rad2/2(ppr)
  Convert pulse to rad2/1(outGearBox) -> outGearBox/1

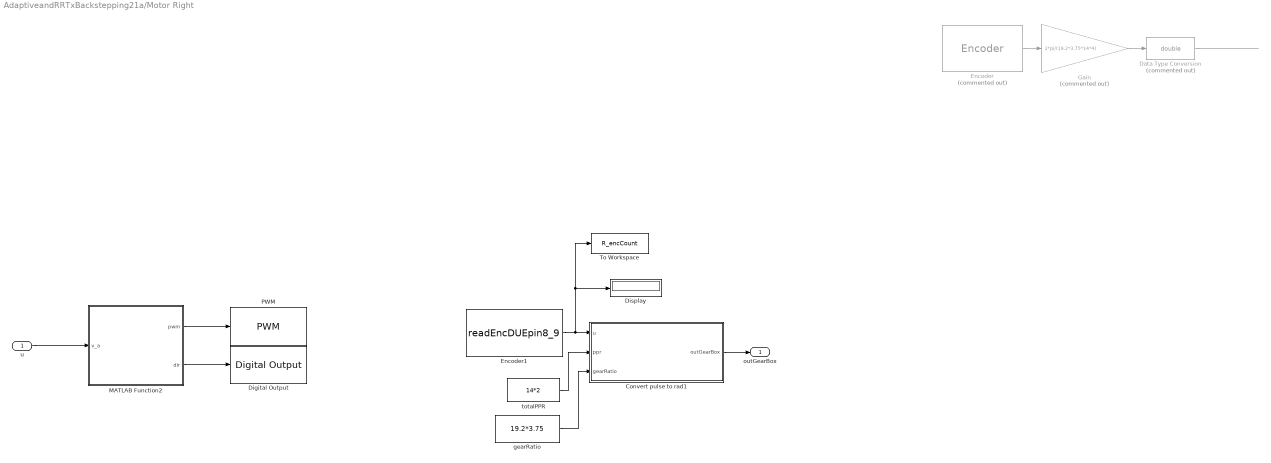
== system AdaptiveandRRTxBackstepping21a/Motor Right ==
  u : Inport
  Convert pulse to rad1 : MATLAB Function  TreatAsAtomicUnit=on
  Data Type Conversion : DataTypeConversion  Commented=on  OutDataTypeStr=double  SaturateOnIntegerOverflow=off  RndMeth=Floor
  Digital Output : arduinolib/Digital Output  pinNumber=7  Direction=output  blockPlatform=arduino
  Display : Display
  Encoder : arduinosensorlib/Encoder  Commented=on  InputA=8  InputB=9  Mode=No reset  SampleTime=-1
      settings: SourceProductBaseCode=ARDUINO
  Encoder1 : S-Function  InitFcn=try, set_param(gcb,'FunctionName','readEncDUEpin8_9'), end  FunctionName=readEncDUEpin8_9  SFunctionModules=readEncDUEpin8_9_wrapper  SFunctionDeploymentMode=off  EnableBusSupport=off  mask(S-Function Builder){}
      mask help: Simulink:masks:SFunctionBuilder_MD
      mask init: same as AdaptiveandRRTxBackstepping21a/Motor Left/Encoder3
      settings: CopyFcn=set_param(gcbh,'LinkStatus','none')  PreSaveFcn=try, set_param(gcb,'FunctionName','readEncDUEpin8_9'), end  OpenFcn=sfunctionwizard(gcbh)
      mask Display:
      | plot(val(:,1),val(:,2))
      | disp(sys)
      | port_label('output',1,'count')
  Gain : Gain  Commented=on  Gain=2*pi/(19.2*3.75*14*4)
  MATLAB Function2 : MATLAB Function  TreatAsAtomicUnit=on
  PWM : arduinolib/PWM  pinNumber=6  frequencyType=Default  desiredFrequency=490.2  achievableFrequency=490.2
  To Workspace : ToWorkspace  VariableName=R_encCount  SaveFormat=Timeseries  SampleTime=-1
  gearRatio : Constant  Value=19.2*3.75
  totalPPR : Constant  Value=14*2
  outGearBox : Outport
  wires:
  MATLAB Function2/1(pwm) -> PWM/1
  MATLAB Function2/2(dir) -> Digital Output/1
  u/1 -> MATLAB Function2/1(v_a)
  gearRatio/1 -> Convert pulse to rad1/3(gearRatio)
  totalPPR/1 -> Convert pulse to rad1/2(ppr)
  Encoder1/1 -> To Workspace/1, Display/1, Convert pulse to rad1/1(u)
  Data Type Conversion/1 -> ?
  Encoder/1 -> Gain/1
  Gain/1 -> Data Type Conversion/1
  Convert pulse to rad1/1(outGearBox) -> outGearBox/1

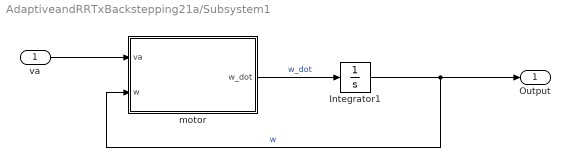
== system AdaptiveandRRTxBackstepping21a/Subsystem1 ==
  va : Inport
  Integrator1 : Integrator
  motor : MATLAB Function  TreatAsAtomicUnit=on
  Output : Outport
  wires:
  Integrator1/1 -> motor/2(w), Output/1  "w"
  motor/1(w_dot) -> Integrator1/1  "w_dot"
  va/1 -> motor/1(va)

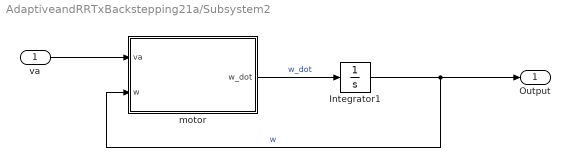
== system AdaptiveandRRTxBackstepping21a/Subsystem2 ==
  va : Inport
  Integrator1 : Integrator
  motor : MATLAB Function  TreatAsAtomicUnit=on
  Output : Outport
  wires:
  Integrator1/1 -> motor/2(w), Output/1  "w"
  motor/1(w_dot) -> Integrator1/1  "w_dot"
  va/1 -> motor/1(va)

== matlab function AdaptiveandRRTxBackstepping21a/controller1 ==
  data: v_d input; w_d input; e1 input; e2 input; e3 input; v_c output; w_c output; V_max input; omega_max input
function [v_c,w_c] =  fcn(v_d, w_d, e1, e2, e3, V_max, omega_max)            

k1 = 4; %1
k2 = 30; %20
k3 = 6; %1
%lambda = 2 ;

% x_e_hat = e1 - k1*w*e2;
% v1 = w*e2 + v_d*cos(e3) - v - k1*w_dot*e2 + k1*w*(w*e1 - v_d*sin(e3));
% v_c = v1 - e2*w + k2*x_e_hat;
% w_c = w_d + lambda*e2*v_d*i + k3*lambda*e3;
%w_c = w_d +k3*lambda*e3;

v_c = k1*e1 + v_d*cos(e3);
w_c = w_d + k2*v_d*e2 + k3*v_d*sin(e3);

if v_c > V_max, v_c = V_max; end
if w_c > omega_max, w_c = omega_max; end

== matlab function AdaptiveandRRTxBackstepping21a/MATLAB Function6 ==
  data: Xd_dot input; v_d output; w_d output
function [v_d, w_d] = fcn(Xd_dot)
% convert velocity in global frame to body frame. No need rotation matrix just need projection.
v_d = sqrt(Xd_dot(1)^2 + Xd_dot(2)^2);
w_d = Xd_dot(3);

== matlab function AdaptiveandRRTxBackstepping21a/f1 ==
  data: theta_d output; x_d input; y_d input
function theta_d = theta( x_d, y_d)
theta_d = zeros(1,length(x_d));
%theta_d(length(x_d)) = 90*pi/180;
for i = 1:length(x_d)-1
       theta_d(i) = atan2(y_d (i+1) - y_d(i), x_d(i+1) - x_d(i));
end

== matlab function AdaptiveandRRTxBackstepping21a/forward kinematic1 ==
  data: v output; w output; theta_c input; fi_R_dot input; X_W_dot output; fi_L_dot input
function [v, w, X_W_dot] = M_inv(theta_c,fi_R_dot, fi_L_dot)
r = 0.07;      %wheel radius r = 0.073
b = 0.42/2   %b = 0.408194/2;

w = r*[0.5/b -0.5/b]*[fi_R_dot; fi_L_dot];
v = r*[0.5 0.5]*[fi_R_dot; fi_L_dot];
X_W_dot = [cos(theta_c) 0;sin(theta_c) 0; 0 1]*[v; w];

== matlab function AdaptiveandRRTxBackstepping21a/MATLAB Function ==
  data: a_hat input; a_dot output; b_hat input; c_hat input; b_dot output; c_dot output; a input; b input; c input
function [a_dot,b_dot,c_dot] = fcn(a_hat,b_hat,c_hat,a,b,c)

lamda = 5;

a_dot = (1/lamda)*(-a+a_hat);
b_dot = (1/lamda)*(-b+b_hat);
c_dot = (1/lamda)*(-c+c_hat);

== matlab function AdaptiveandRRTxBackstepping21a/invers Rotation Matrix (R(fi))1 ==
  data: e_w input; theta_c input; e_R output
function e_R = fcn(e_w,theta_c)
%#codegen

R = [cos(theta_c), sin(theta_c), 0; -sin(theta_c), cos(theta_c), 0; 0, 0, 1]; % to substract theta, origin of desired theta frame and current theta need to be the same, although they are both respect to global frame but they could have different origin sometimes. 
e_R = R*e_w;

== matlab function AdaptiveandRRTxBackstepping21a/MATLAB Function7 ==
  settings: updateMethod=DISCRETE
  data: t input; route input; x_d input; y_d input; theta_d input; X_r_dot output; X input; V_max output; omega_max output; X_W_c input
function [X_r_dot, V_max, omega_max]   = fcn(t,route,x_d,y_d,theta_d, X, X_W_c)
%#codegen

persistent k i j X_p_i omega_p_j t1 t2
if isempty(k)
    i = int8(1);
    j = int8(1);
    X_p_i = [0;0];
    omega_p_j = 0;
    t1 = t;
    t2 = t;
    k = 1;
end
tau = 0.15;
tau1 = 0.15;
V_max = 0.2; % maximum velocity0.2
a = 5;      % acceleration0.1
omega_max = 2; %0.15
alpha = 1; %0.1

X_r_dot = zeros(3,1);
switch route
    case 1
%         X_p = [1.5   1.5  0];
%%%%%%%%%%%%%theta_d = zeros(length(x),1);
        X_p = [x_d,y_d,theta_d]; % X_p = [x,y,theta];
    otherwise
        X_r_dot = [0;0;0];
        return;
end
X_p = X_p'; % X_p = [x;y;theta]
[~,col] = size(X_p);
dX = X_p(1:2,i)-X_p_i;
norm_dX = norm(dX);
two_rmin = V_max^2/a;  
dtheta = X_p(3,j)-omega_p_j;
norm_dtheta = abs(dtheta);
two_thetamin = omega_max^2/alpha; 

if norm_dX > two_rmin
    ta = V_max/a;                   % acceleration period
    tad = (norm_dX-two_rmin)/V_max; % acc to deceleration period
    td = ta + tad;                  % start deceleration
    te = ta + td;                   % end deceleration
    if (t-t1) < ta
        v = a*(t-t1);
    elseif ta <= (t-t1) && (t-t1) < td
        v = V_max;
    elseif td <= (t-t1) && (t-t1) < te
        v = -a*(t-t1-td) + V_max;
    else
        v = 0;
    end
else
    tp = sqrt(norm_dX/a);
    te = 2*tp;
    Vp = a*tp;
    if (t-t1) < tp
        v = a*(t-t1);
    elseif tp < (t-t1) && (t-t1) < te
        v = -a*(t-t1-tp)+Vp;
    else
        v = 0;
    end
end
if norm_dX~=0
    X_r_dot(1:2) = v*dX/norm_dX;
end

dist_X = norm(X_p(1:2,i)-X(1:2));
if (i<col)&&(dist_X < tau)
    X_p_i = X(1:2);
    t1    = t;
    i     = i+1;
end

if norm_dtheta > two_thetamin
    ta = omega_max/alpha;                   % acceleration period
    tad = (norm_dtheta-two_thetamin)/omega_max; % acc to deceleration period
    td = ta + tad;                  % start deceleration
    te = ta + td;                   % end deceleration
    if (t-t2) < ta
        omega = alpha*(t-t2);
    elseif ta <= (t-t2) && (t-t2) < td
        omega = omega_max;
    elseif td <= (t-t2) && (t-t2) < te
        omega = -alpha*(t-t2-td) + omega_max;
    else
        omega = 0;
    end
else
    tp = sqrt(norm_dtheta/alpha);
    te = 2*tp;
    omegap = alpha*tp;
    if (t-t2) < tp
        omega = alpha*(t-t2);
    elseif tp < (t-t2) && (t-t2) < te
        omega = -alpha*(t-t2-tp)+omegap;
    else
        omega = 0;
    end
end
X_r_dot(3) = omega*sign(dtheta);

%Generate w to control final point orientation
e_x = abs(X_W_c(1) - X_p(1,end));
e_y = abs(X_W_c(2) - X_p(2,end));
e_theta = X_W_c(3) - X_p(3,end);
if  e_x < 0.5 && e_y < 0.5 && abs(e_theta) > 3*pi/180
    omega = -2*(X_W_c(3) - X_p(3,end));
elseif e_x < 0.5 && e_y < 0.5 && abs(e_theta) <= 3*pi/180
    omega = 0;
end
X_r_dot(3) = omega;

dist_theta = abs(X_p(3,j)-X(3));
if (j<col)&&(dist_theta < tau1)
    omega_p_j = X(3);
    t2    = t;
    j     = j+1;
end

== matlab function AdaptiveandRRTxBackstepping21a/controller3 ==
  data: v_d input; w_d input; e1 input; e2 input; e3 input; v_c output; w_c output; V_max input; omega_max input
function [v_c,w_c] =  fcn(v_d, w_d, e1, e2, e3, V_max, omega_max)            

k1 = 4; %1
k2 = 30; %20
k3 = 6; %1
%lambda = 2 ;

% x_e_hat = e1 - k1*w*e2;
% v1 = w*e2 + v_d*cos(e3) - v - k1*w_dot*e2 + k1*w*(w*e1 - v_d*sin(e3));
% v_c = v1 - e2*w + k2*x_e_hat;
% w_c = w_d + lambda*e2*v_d*i + k3*lambda*e3;
%w_c = w_d +k3*lambda*e3;

v_c = k1*e1 + v_d*cos(e3);
w_c = w_d + k2*v_d*e2 + k3*v_d*sin(e3);

if v_c > V_max, v_c = V_max; end
if w_c > omega_max, w_c = omega_max; end

== matlab function AdaptiveandRRTxBackstepping21a/f2 ==
  data: theta_d output; x_d input; y_d input
function theta_d = theta( x_d, y_d)
theta_d = zeros(1,length(x_d));
%theta_d(length(x_d)) = 220*pi/180;
for i = 1:length(x_d)-1
       theta_d(i) = atan2(y_d (i+1) - y_d(i), x_d(i+1) - x_d(i));
end

== matlab function AdaptiveandRRTxBackstepping21a/forward kinematic4 ==
  data: v output; w output; theta_c input; fi_R_dot input; X_W_dot output; fi_L_dot input
function [v, w, X_W_dot] = M_inv(theta_c,fi_R_dot, fi_L_dot)
r = 0.07;      %wheel radius
b = 0.21; 

w = r*[0.5/b -0.5/b]*[fi_R_dot; fi_L_dot];
v = r*[0.5 0.5]*[fi_R_dot; fi_L_dot];
X_W_dot = [cos(theta_c) 0;sin(theta_c) 0; 0 1]*[v; w];

== matlab function AdaptiveandRRTxBackstepping21a/invers Rotation Matrix (R(fi))4 ==
  data: e_w input; theta_c input; e_R output
function e_R = fcn(e_w,theta_c)
%#codegen

R = [cos(theta_c), sin(theta_c), 0; -sin(theta_c), cos(theta_c), 0; 0, 0, 1]; % to substract theta, origin of desired theta frame and current theta need to be the same, although they are both respect to global frame but they could have different origin sometimes. 
e_R = R*e_w;

== matlab function AdaptiveandRRTxBackstepping21a/invers kinematic4 ==
  data: v input; fi_R_dot output; w input; fi_L_dot output
function [fi_R_dot, fi_L_dot] = M_inv(v, w)
r = 0.07;      %wheel radius
b = 0.21; 
fi_R_dot = (v + w*b)/r;
fi_L_dot = (v - w*b)/r;

== matlab function AdaptiveandRRTxBackstepping21a/invers kinematic1 ==
  data: v input; fi_R_dot output; w input; fi_L_dot output
function [fi_R_dot, fi_L_dot] = M_inv(v, w)
r = 0.07;      %wheel radius r = 0.073
b = 0.42/2   %b = 0.408194/2;

fi_R_dot = (v + w*b)/r;
fi_L_dot = (v - w*b)/r;

== matlab function AdaptiveandRRTxBackstepping21a/MATLAB Function10 ==
  data: comp output; one_on_b output; a input; a_on_b output; b input; c input; w input; kp output; ki output
function [comp,one_on_b,a_on_b,kp,ki] = fcn(a,b,c,w)

a_on_b = (a/b)*w;
one_on_b = (1/b)*w;
comp = (c/b)*sign(w);

wn = 2*pi*6;
zeta = 1;

ki = wn^2/b;
kp = (2*zeta*wn-a)/b;

== matlab function AdaptiveandRRTxBackstepping21a/MATLAB Function11 ==
  settings: updateMethod=DISCRETE
  data: x_pre input; P_pre input; y_true input; x output; uk input; P output
function [x,P] = ekf(x_pre,P_pre,y_true, uk)
Ts = 0.01;

Qc_est  = 1e-4*diag([1,10,10,10]);
Qd_est  = Ts*Qc_est;
R_est   = 0.01;

Ck = [1 0 0 0];
Dk = 0;


% PREDICTION STEP
%Compute prediction at next time step
x = x_pre+Ts*[-x_pre(2)*x_pre(1) + uk*x_pre(3) - x_pre(4)*sign(x_pre(1));
                0;
                0;
                0];

Ak = eye(4)+Ts*[-x_pre(2) -x_pre(1) uk -sign(x_pre(1));
                 0     0    0      0;
                 0     0    0      0;
                 0     0    0      0];
P = Ak*P_pre*Ak'+Qd_est;

% OBSERVATION AND UPDATE
%Comput Kalman Gain and update predicted value
Wk    = P*Ck'/(Ck*P*Ck'+R_est);
y_est = Ck*x+Dk*uk;
dely = y_true-y_est;
Wkdely = Wk*dely;
x = x+Wkdely;
P = P-Wk*Ck*P;

== matlab function AdaptiveandRRTxBackstepping21a/MATLAB Function12 ==
  data: comp output; one_on_b output; a input; a_on_b output; b input; c input; w input; kp output; ki output
function [comp,one_on_b,a_on_b,kp,ki] = fcn(a,b,c,w)

a_on_b = (a/b)*w;
one_on_b = (1/b)*w;
comp = (c/b)*sign(w);

wn = 2*pi*6;
zeta = 1;

ki = wn^2/b;
kp = (2*zeta*wn-a)/b;

== matlab function AdaptiveandRRTxBackstepping21a/MATLAB Function13 ==
  settings: updateMethod=DISCRETE
  data: x_pre input; P_pre input; y_true input; x output; uk input; P output
function [x,P] = ekf(x_pre,P_pre,y_true, uk)
Ts = 0.01;

Qc_est  = 1e-4*diag([1,10,10,10]);
Qd_est  = Ts*Qc_est;
R_est   = 0.01;

Ck = [1 0 0 0];
Dk = 0;


% PREDICTION STEP
%Compute prediction at next time step
x = x_pre+Ts*[-x_pre(2)*x_pre(1) + uk*x_pre(3) - x_pre(4)*sign(x_pre(1));
                0;
                0;
                0];

Ak = eye(4)+Ts*[-x_pre(2) -x_pre(1) uk -sign(x_pre(1));
                 0     0    0      0;
                 0     0    0      0;
                 0     0    0      0];
P = Ak*P_pre*Ak'+Qd_est;

% OBSERVATION AND UPDATE
%Comput Kalman Gain and update predicted value
Wk    = P*Ck'/(Ck*P*Ck'+R_est);
y_est = Ck*x+Dk*uk;
dely = y_true-y_est;
Wkdely = Wk*dely;
x = x+Wkdely;
P = P-Wk*Ck*P;

== matlab function AdaptiveandRRTxBackstepping21a/MATLAB Function5 ==
  data: a output; b output; c output; t input; a_nw input; b_nw input; c_nw input
function [a,b,c] = fcn(t,a_nw,b_nw,c_nw)             


a = 28.37;
b = 19.15;
c = 5.75;


if t>0.5
a = a_nw;
b = b_nw;
c = c_nw;
end

== matlab function AdaptiveandRRTxBackstepping21a/MATLAB Function8 ==
  data: a_hat input; a_dot output; b_hat input; c_hat input; b_dot output; c_dot output; a input; b input; c input
function [a_dot,b_dot,c_dot] = fcn(a_hat,b_hat,c_hat,a,b,c)

lamda = 5;

a_dot = (1/lamda)*(-a+a_hat);
b_dot = (1/lamda)*(-b+b_hat);
c_dot = (1/lamda)*(-c+c_hat);

== matlab function AdaptiveandRRTxBackstepping21a/MATLAB Function9 ==
  data: a output; b output; c output; t input; a_nw input; b_nw input; c_nw input
function [a,b,c] = fcn(t,a_nw,b_nw,c_nw)             


a = 26.63;
b = 17.26;
c = 6.776;


if t>0.5
a = a_nw;
b = b_nw;
c = c_nw;
end

== matlab function AdaptiveandRRTxBackstepping21a/Motor Left/Convert pulse to rad2 ==
  settings: updateMethod=DISCRETE
  data: u input; ppr input; gearRatio input; outGearBox output
function outGearBox = fcn(u,ppr,gearRatio)

persistent counter_num over_flag
if(isempty(counter_num)), counter_num = 0;end
if(isempty(over_flag)), over_flag = 0;end
pulse2radian = 2*pi/ppr; % 1 pulse = ?? radian

if(double(u) - counter_num > 40000), over_flag = over_flag-1;
elseif(double(u) - counter_num < -40000), over_flag = over_flag+1;
end

inGearBox = (double(u)+over_flag*(2^32 -1))*pulse2radian; 
outGearBox = inGearBox/gearRatio;
counter_num = double(u) ;

== matlab function AdaptiveandRRTxBackstepping21a/MATLAB Function14 ==
  data: a_hat input; a_dot output; b_hat input; c_hat input; b_dot output; c_dot output; a input; b input; c input
function [a_dot,b_dot,c_dot] = fcn(a_hat,b_hat,c_hat,a,b,c)

lamda = 4;

a_dot = (1/lamda)*(-a+a_hat);
b_dot = (1/lamda)*(-b+b_hat);
c_dot = (1/lamda)*(-c+c_hat);

== matlab function AdaptiveandRRTxBackstepping21a/Motor Left/MATLAB Function3 ==
  data: v_a input; pwm output; dir output
function [pwm,dir] = fcn(v_a)

vmax = 22.5;
pwm_cal = v_a*254/vmax;
if pwm_cal > 0
    pwm = pwm_cal;
    dir = 1;
elseif pwm_cal < 0
    pwm = abs(pwm_cal);
    dir = 0;
else
    pwm = 0;
    dir = 0;
end

== matlab function AdaptiveandRRTxBackstepping21a/Motor Right/Convert pulse to rad1 ==
  settings: updateMethod=DISCRETE
  data: u input; ppr input; gearRatio input; outGearBox output
function outGearBox = fcn(u,ppr,gearRatio)

persistent counter_num over_flag
if(isempty(counter_num)), counter_num = 0;end
if(isempty(over_flag)), over_flag = 0;end
pulse2radian = 2*pi/ppr; % 1 pulse = ?? radian

if(double(u) - counter_num > 40000), over_flag = over_flag-1;
elseif(double(u) - counter_num < -40000), over_flag = over_flag+1;
end

inGearBox = (double(u)+over_flag*(2^32 -1))*pulse2radian; 
outGearBox = inGearBox/gearRatio;
counter_num = double(u) ;

== matlab function AdaptiveandRRTxBackstepping21a/Motor Right/MATLAB Function2 ==
  data: v_a input; pwm output; dir output
function [pwm,dir] = fcn(v_a)

vmax = 22.5;
pwm_cal = (v_a*254/vmax);
if pwm_cal > 0
    pwm = pwm_cal;
    dir = 0;
elseif pwm_cal < 0
    pwm = abs(pwm_cal);
    dir = 1;
else
    pwm = 0;
    dir = 0;
end

== matlab function AdaptiveandRRTxBackstepping21a/MATLAB Function18 ==
  data: comp output; one_on_b output; a input; a_on_b output; b input; c input; w input; kp output; ki output
function [comp,one_on_b,a_on_b,kp,ki] = fcn(a,b,c,w)

a_on_b = (a/b)*w;
one_on_b = (1/b)*w;
comp = (c/b)*sign(w);

wn = 2*pi*6;
zeta = 1;

ki = wn^2/b;
kp = (2*zeta*wn-a)/b;

== matlab function AdaptiveandRRTxBackstepping21a/MATLAB Function19 ==
  settings: updateMethod=DISCRETE
  data: uk input; y_true input; x_est output
function x_est = ekf(uk,y_true)
Ts = 0.01;
persistent x_est_p P Qd_est R_est Qc_est;
if isempty(x_est_p)
    x_est_p = [0;0;0;0];
    P       = 1e-0*diag([10,1,30,1]);
    Qc_est  = 1e-4*diag([1,10,100,10]);
    Qd_est  = Ts*Qc_est;
    R_est   = 0.001;
end
c  = [1 0 0 0];
D  = 0;
Ck = c;
Dk = D;

%Comput Kalman Gain and update predicted value
Wk    = P*Ck'/(Ck*P*Ck'+R_est);
y_est = Ck*x_est_p+Dk*uk;
x     = x_est_p+Wk.*(y_true-y_est);

%Compute prediction at next time step
x_est = x+Ts*[-x(2)*x(1)+uk*x(3)-x(4)*sign(x(1));
                          0;
                          0;
                          0];

%Update error covariance matrices
P = P-Wk*Ck*P;

%Define Ak
Ak      = eye(4)+Ts*[-x(2) -x(1) uk -sign(x(1));
                 0     0    0      0;
                 0     0    0      0;
                 0     0    0      0];
P       = Ak*P*Ak'+Qd_est;
x_est_p = x_est;

== matlab function AdaptiveandRRTxBackstepping21a/MATLAB Function22 ==
  data: a_hat input; a_dot output; b_hat input; c_hat input; b_dot output; c_dot output; a input; b input; c input
function [a_dot,b_dot,c_dot] = fcn(a_hat,b_hat,c_hat,a,b,c)

lamda = 4;

a_dot = (1/lamda)*(-a+a_hat);
b_dot = (1/lamda)*(-b+b_hat);
c_dot = (1/lamda)*(-c+c_hat);

== matlab function AdaptiveandRRTxBackstepping21a/MATLAB Function23 ==
  data: a output; b output; c output; t input; a_nw input; b_nw input; c_nw input
function [a,b,c] = fcn(t,a_nw,b_nw,c_nw)

a = 26.63;
b = 17.26;
c = 6.776;

if t>0.5
a = a_nw;
b = b_nw;
c = c_nw;
end

== matlab function AdaptiveandRRTxBackstepping21a/Subsystem1/motor ==
  data: va input; w_dot output; w input
function w_dot = fcn(va, w)
a = 28.37;
b = 19.15;
c = 5.75;

w_dot = -a*w+b*va-c*sign(w);

== matlab function AdaptiveandRRTxBackstepping21a/Subsystem2/motor ==
  data: va input; w_dot output; w input
function w_dot = fcn(va, w)
a = 26.63;
b = 17.26;
c = 6.776;

w_dot = -a*w+b*va-c*sign(w);

== matlab function AdaptiveandRRTxBackstepping21a/MATLAB Function15 ==
  data: comp output; one_on_b output; a input; a_on_b output; b input; c input; w input; kp output; ki output
function [comp,one_on_b,a_on_b,kp,ki] = fcn(a,b,c,w)

a_on_b = (a/b)*w;
one_on_b = (1/b)*w;
comp = (c/b)*sign(w);

wn = 2*pi*6;
zeta = 1;

ki = wn^2/b;
kp = (2*zeta*wn-a)/b;
